simulink model "UAV4"  (R2022b)
settings: Solver=FixedStepAuto  StartTime=0  StopTime=1000000  FixedStep=0.01  RelTol=1e-3
libraries: uavalgslib x2, robotcorelib x1, uavutilslib x1
settings Model: DataDictionary=fixedWingPathFollowingData.sldd  EnableAccessToBaseWorkspace=off  SimulationMode=accelerator  NumberOfSteps=1000  PacingRate=10  Creator=The MathWorks, Inc.  LastModifiedBy=Amruth
settings SolverCC: AlgebraicLoopSolver=TrustRegion  DecoupledContinuousIntegration=on
settings DataIOCC: ReturnWorkspaceOutputs=off
settings DebuggingCC: UnconnectedInputMsg=warning  UnconnectedOutputMsg=warning  UnconnectedLineMsg=warning  SFMachineParentedDataDiag=warning  ArithmeticOperatorsInVariantConditions=warning
settings ModelReferenceCC: EnableRefExpFcnMdlSchedulingChecks=on
settings SFSimCC: SimUseLocalCustomCode=off  CustomCodeUndefinedFunction=UseInterfaceOnly
settings RTWCC: RTWUseLocalCustomCode=off  DLArmComputeVersion=19.05

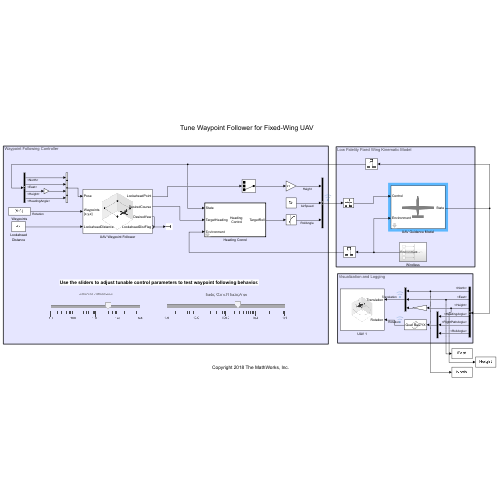
[thumbnail: Simulink's stored preview of the top-level diagram]
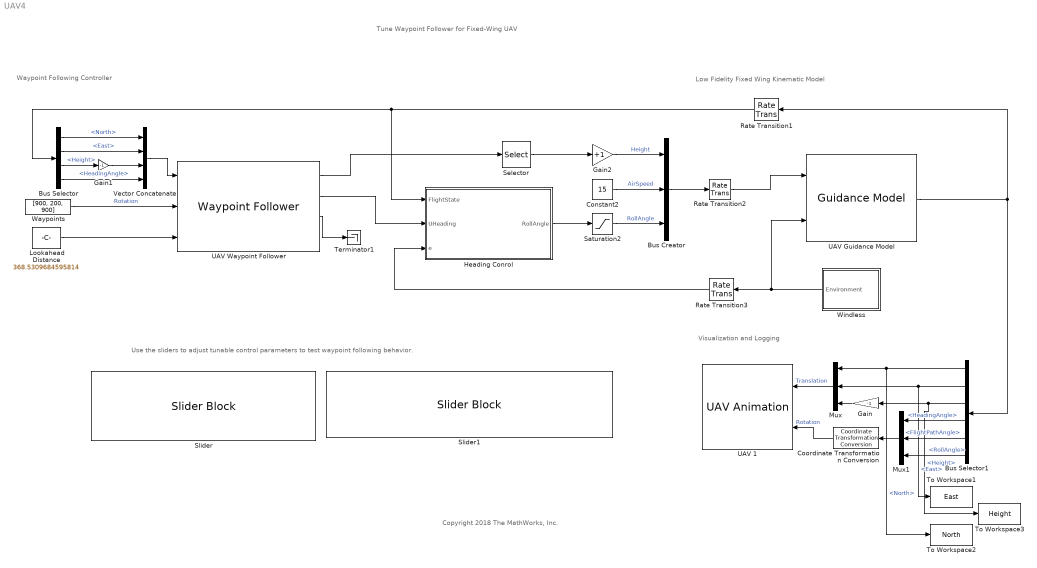
== system UAV4 ==
  note: Tune Waypoint Follower for Fixed-Wing UAV
  note: Use the sliders to adjust tunable control parameters to test waypoint following behavior.
  note: Visualization and Logging
  note: Low Fidelity Fixed Wing Kinematic Model
  note: Waypoint Following Controller
  note: Copyright 2018 The MathWorks, Inc.
  Bus Creator : BusCreator  Inputs=3  OutDataTypeStr=Bus: FixedWingControlBus  NonVirtualBus=on
  Bus Selector : BusSelector  OutputSignals=North,East,Height,HeadingAngle
  Bus Selector1 : BusSelector  OutputSignals=North,East,Height,HeadingAngle,FlightPathAngle,RollAngle
  Constant2 : Constant  Value=15
  Coordinate Transformation Conversion : robotcorelib/Coordinate Transformation Conversion  InputRepresentation=Euler Angles  InputEulerSequence=ZYX  ShowTrVecInputPort=on  OutputRepresentation=Quaternion  OutputEulerSequence=ZYX  ShowTrVecOutputPort=on  SimulateUsing=Code generation
  Gain : Gain  Gain=-1
  Gain1 : Gain  Gain=-1
  Gain2 : Gain  Gain=+1
  Heading Conrol : MATLAB Function  TreatAsAtomicUnit=on  mask(Fixed Wing Heading Controller){PHeadingAngle=257.3240329601091}
      mask prompts: PHeadingAngle "Heading Control Gain"
      mask help: P controller that regulates fixed wing UAV heading direction through controlling its roll angle. This controller requires that the plane is flying under coordinated flight condition.
  Lookahead Distance : Constant  Value=368.5309684595814
  Mux : Mux  Inputs=3
  Mux1 : Mux  Inputs=3
  Rate Transition1 : RateTransition  OutPortSampleTime=0.01
  Rate Transition2 : RateTransition  OutPortSampleTime=0.1
  Rate Transition3 : RateTransition  OutPortSampleTime=0.01
  Saturation2 : Saturate  UpperLimit=20/180*pi  LowerLimit=-20/180*pi
  Selector : Selector  InputPortWidth=3  IndexOptions=Index vector (dialog)  Indices=[3]  OutputSizes=1
  Slider : SliderBlock  ScaleMin=1  ScaleMax=10000  ScaleType=Log
  Slider1 : SliderBlock  ScaleMin=1  ScaleMax=10000  ScaleType=Log
  Terminator1 : Terminator
  To Workspace1 : ToWorkspace  VariableName=East  SampleTime=-1
      settings: Save2DSignal=2-D array (concatenate along first dimension)
  To Workspace2 : ToWorkspace  VariableName=North  SampleTime=-1
      settings: Save2DSignal=2-D array (concatenate along first dimension)
  To Workspace3 : ToWorkspace  VariableName=Height  SampleTime=-1
      settings: Save2DSignal=2-D array (concatenate along first dimension)
  UAV 1 : uavutilslib/UAV Animation  UAVType=Multirotor  UAVSize=50  InertialZDirection=Down  SampleTime=-1
  UAV Guidance Model : uavalgslib/Guidance Model  ModelType=FixedWingGuidance  SpecifiedDataType=double  SimulateUsing=Interpreted execution  InitialWorldPositionMultirotor=[0; 0; 0]  InitialWorldVelocityMultirotor=[0; 0; 0]  InitialEulerZYXMultirotor=[0; 0; 0]  InitialBodyAngularRateRPYMultirotor=[0; 0; 0]  InitialThrustMultirotor=0  InitialNorthFixedWing=800  InitialEastFixedWing=600  InitialHeightFixedWing=0  InitialAirSpeedFixedWing=15  InitialHeadingAngleFixedWing=180  InitialFlightPathAngleFixedWing=0  InitialRollAngleFixedWing=800  InitialRollAngleRateFixedWing=0  PDRollMultirotor=[3402.97,116.67]  PDPitchMultirotor=[3402.97, 116.67]  PYawRateMultirotor=1950  PThrustMultirotor=3900  MassMultirotor=0.1  PHeightFixedWing=80  PHeadingAngleFixedWing=3.9  PFlightPathAngleFixedWing=80  PDRollFixedWing=[5.9414, 3.9]  PAirSpeedFixedWing=1  FlightPathAngleLimitsFixedWing=[-pi/6, pi/6]  StateBusName='FixedWingStateBus'  ControlBusName='FixedWingControlBus'  EnvironmentBusName='FixedWingEnvironmentBus'  DataType=double
  UAV Waypoint Follower : uavalgslib/Waypoint Follower  UAVType=fixed-wing  StartFrom=first  TransitionRadiusSource=internal  TransitionRadius=10  MinLookaheadDistance=0.1  YawInput=off  ShowCrossTrackErrorOutput=off  ShowStatusOutput=off  SimulateUsing=Code generation
  Vector Concatenate : Concatenate  NumInputs=4
  Waypoints : Constant  Value=[900, 200, 900]  VectorParams1D=off
  Windless : Subsystem  VariantControl=NoWind
  wires:
  Constant2/1 -> Bus Creator/2  "AirSpeed"
  Gain2/1 -> Bus Creator/1  "Height"
  Bus Creator/1 -> Rate Transition2/1
  Bus Selector/1 -> Vector Concatenate/1  "<North>"
  Bus Selector/2 -> Vector Concatenate/2  "<East>"
  Saturation2/1 -> Bus Creator/3  "RollAngle"
  Rate Transition1/1 -> Heading Conrol/1(FlightState), Bus Selector/1
  Rate Transition2/1 -> UAV Guidance Model/1
  UAV Waypoint Follower/2 -> Heading Conrol/2(UHeading)
  UAV Waypoint Follower/1 -> Selector/1
  Vector Concatenate/1 -> UAV Waypoint Follower/1
  UAV Waypoint Follower/3 -> Terminator1/1
  Lookahead Distance/1 -> UAV Waypoint Follower/3
  Heading Conrol/1(RollAngle) -> Saturation2/1
  Gain/1 -> Mux/3
  Bus Selector1/6 -> Mux1/3  "<RollAngle>"
  Bus Selector1/5 -> Mux1/2  "<FlightPathAngle>"
  Mux1/1 -> Coordinate Transformation Conversion/1
  Coordinate Transformation Conversion/1 -> UAV 1/2  "Rotation"
  UAV Guidance Model/1 -> Bus Selector1/1, Rate Transition1/1
  Mux/1 -> UAV 1/1  "Translation"
  Windless/1(Environment) -> UAV Guidance Model/2, Rate Transition3/1
  Bus Selector/4 -> Vector Concatenate/4  "<HeadingAngle>"
  Bus Selector/3 -> Gain1/1  "<Height>"
  Gain1/1 -> Vector Concatenate/3
  Selector/1 -> Gain2/1
  Rate Transition3/1 -> Heading Conrol/3(e)
  Bus Selector1/1 -> To Workspace2/1, Mux/1  "<North>"
  Bus Selector1/2 -> Mux/2, To Workspace1/1  "<East>"
  Bus Selector1/4 -> Mux1/1  "<HeadingAngle>"
  Bus Selector1/3 -> To Workspace3/1, Gain/1  "<Height>"
  Waypoints/1 -> UAV Waypoint Follower/2  "Rotation"

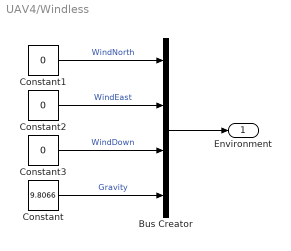
== system UAV4/Windless ==
  Bus Creator : BusCreator  Inputs=4  OutDataTypeStr=Bus: FixedWingEnvironmentBus  NonVirtualBus=on
  Constant : Constant  Value=9.8066
  Constant1 : Constant  Value=0
  Constant2 : Constant  Value=0
  Constant3 : Constant  Value=0
  Environment : Outport  VectorParamsAs1DForOutWhenUnconnected=off
  wires:
  Constant2/1 -> Bus Creator/2  "WindEast"
  Constant3/1 -> Bus Creator/3  "WindDown"
  Constant1/1 -> Bus Creator/1  "WindNorth"
  Bus Creator/1 -> Environment/1
  Constant/1 -> Bus Creator/4  "Gravity"

== matlab function UAV4/Heading Conrol ==
  data: FlightState input; UHeading input; RollAngle output size=[1 1]; e input; PHeadingAngle parameter
function RollAngle = fcn(FlightState, UHeading, e, PHeadingAngle)
    
    Va = FlightState.AirSpeed;
    HeadingAngle = FlightState.HeadingAngle;
    FlightPathAngle = FlightState.FlightPathAngle;
    
    YawAngle = HeadingAngle - asin((1/Va)*[e.WindNorth, e.WindEast]*[-sin(HeadingAngle); cos(HeadingAngle)]);
    b = [cos(HeadingAngle)*cos(FlightPathAngle), sin(HeadingAngle)*cos(FlightPathAngle), -sin(FlightPathAngle)]*[e.WindNorth; e.WindEast; e.WindDown];
    c = [e.WindNorth, e.WindEast, e.WindDown]*[e.WindNorth; e.WindEast; e.WindDown]- Va^2;
    Vg = -b+sqrt(b^2-c);
    
    RollAngle = atan2(PHeadingAngle*angdiff(HeadingAngle,UHeading)*Vg,e.Gravity*cos(HeadingAngle-YawAngle));
